simulink model "braking_ABS_Fin"  (Simulink 8.5)
settings: Solver=ode45  StartTime=0.0  StopTime=7  MaxStep=0.05  RelTol=1e-5
values from neighbouring files (symbols this model uses):
  Iw = 1    [Inizializza.m]
  M = 1500/4    (= 375)    [Inizializza.m]
  mu = [0 0.45 0.9 0.8 0.65]'    [Inizializza.m]
  Rw = 0.3    [Inizializza.m]
  slip = [0 0.1 0.2 0.6 1]'    [Inizializza.m]
  Tbmax = 1500    [Inizializza.m]
  V0 = 100/3.6    (= 27.7777777778)    [Inizializza.m]
libraries: simulink x3
settings Model: Creator=Domenico  LastModifiedBy=utente
settings DebuggingCC: SolverPrmCheckMsg=warning  FcnCallInpInsideContextMsg=UseLocalSettings

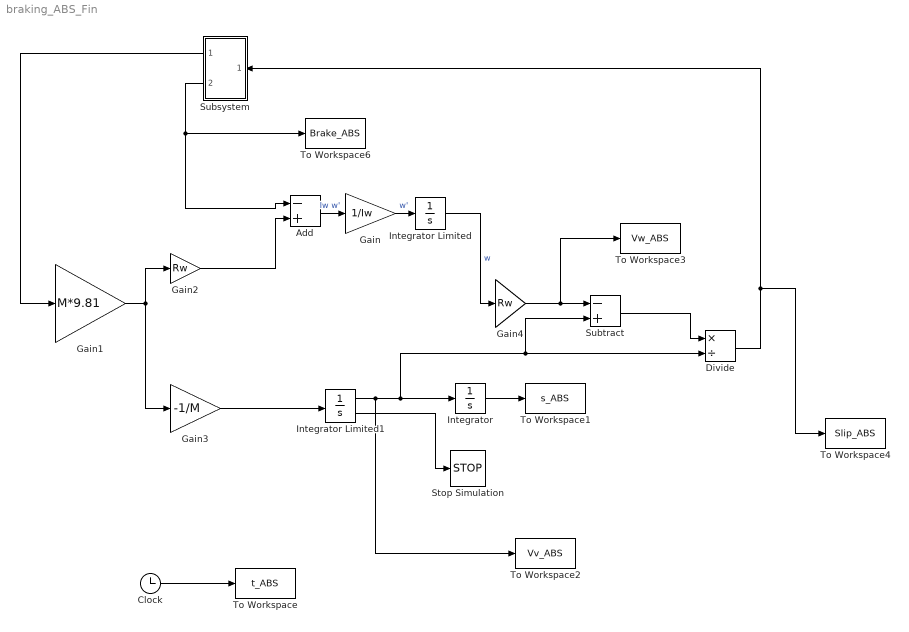
== system braking_ABS_Fin ==
  Add : Sum  Inputs=-+
  Clock : Clock
  Divide : Product  Inputs=*/
  Gain : Gain  Gain=1/Iw
  Gain1 : Gain  Gain=M*9.81
  Gain2 : Gain  Gain=Rw
  Gain3 : Gain  Gain=-1/M
  Gain4 : Gain  Gain=Rw
  Integrator : Integrator
  Integrator Limited : Integrator  InitialCondition=V0/Rw  LimitOutput=on  UpperSaturationLimit=2*V0/Rw  LowerSaturationLimit=0
  Integrator Limited1 : Integrator  InitialCondition=V0  LimitOutput=on  UpperSaturationLimit=2*V0  LowerSaturationLimit=0.5  ShowSaturationPort=on
  Stop Simulation : Stop
  Subsystem : Subsystem
  Subtract : Sum  Inputs=-+
  To Workspace : ToWorkspace  VariableName=t_ABS  SampleTime=-1
  To Workspace1 : ToWorkspace  VariableName=s_ABS  SampleTime=-1
  To Workspace2 : ToWorkspace  VariableName=Vv_ABS  SampleTime=-1
  To Workspace3 : ToWorkspace  VariableName=Vw_ABS  SampleTime=-1
  To Workspace4 : ToWorkspace  VariableName=Slip_ABS  SampleTime=-1
  To Workspace6 : ToWorkspace  VariableName=Brake_ABS  SampleTime=-1
  wires:
  Add/1 -> Gain/1  "Iw w'"
  Gain/1 -> Integrator Limited/1  "w'"
  Integrator Limited/1 -> Gain4/1  "w"
  Gain2/1 -> Add/2
  Gain3/1 -> Integrator Limited1/1
  Integrator Limited1/2 -> Stop Simulation/1
  Integrator Limited1/1 -> Integrator/1, Subtract/2, Divide/2, To Workspace2/1
  Integrator/1 -> To Workspace1/1
  Gain4/1 -> Subtract/1, To Workspace3/1
  Subtract/1 -> Divide/1
  Divide/1 -> Subsystem/1(In1), To Workspace4/1
  Subsystem/1(Out1) -> Gain1/1
  Gain1/1 -> Gain2/1, Gain3/1
  Subsystem/2(Out2) -> Add/1, To Workspace6/1
  Clock/1 -> To Workspace/1

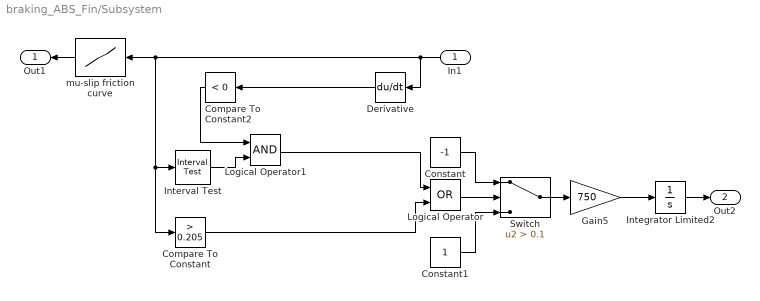
== system braking_ABS_Fin/Subsystem ==
  In1 : Inport
  Compare To Constant : simulink/Logic and Bit Operations/Compare To Constant  relop=>  const=0.205  OutDataTypeStr=uint8
  Compare To Constant2 : simulink/Logic and Bit Operations/Compare To Constant  relop=<  const=0  OutDataTypeStr=uint8
  Constant : Constant  Value=-1
  Constant1 : Constant
  Derivative : Derivative
  Gain5 : Gain  Gain=750
  Integrator Limited2 : Integrator  LimitOutput=on  UpperSaturationLimit=Tbmax  LowerSaturationLimit=0
  Interval Test : simulink/Logic and Bit Operations/Interval Test  IntervalClosedRight=on  uplimit=0.195  IntervalClosedLeft=on  lowlimit=0.19  OutDataTypeStr=boolean
  Logical Operator : Logic  Operator=OR  AllPortsSameDT=off  OutDataTypeStr=boolean
  Logical Operator1 : Logic  AllPortsSameDT=off  OutDataTypeStr=boolean
  Switch : Switch  Criteria=u2 > Threshold  Threshold=0.1
  mu-slip friction curve : Lookup  InputValues=slip  Table=mu  SaturateOnIntegerOverflow=on
  Out1 : Outport
  Out2 : Outport  Port=2
  wires:
  Switch/1 -> Gain5/1
  Gain5/1 -> Integrator Limited2/1
  Constant/1 -> Switch/1
  Constant1/1 -> Switch/3
  Compare To Constant/1 -> Logical Operator/2
  Logical Operator/1 -> Switch/2
  Interval Test/1 -> Logical Operator1/2
  Derivative/1 -> Compare To Constant2/1
  Compare To Constant2/1 -> Logical Operator1/1
  Logical Operator1/1 -> Logical Operator/1
  In1/1 -> mu-slip friction curve/1, Compare To Constant/1, Interval Test/1, Derivative/1
  mu-slip friction curve/1 -> Out1/1
  Integrator Limited2/1 -> Out2/1
